simulink model "fuz_model"  (R2018a)
settings: Solver=VariableStepAuto  StartTime=0.0  StopTime=inf  RelTol=1e-3
undefined symbols (not defined in the file): DeltaDVal, DeltaIVal, DeltaPVal
libraries: robotlib x5, fuzblock x1
settings Model: Creator=piradata  LastModifiedBy=piradata
settings DataIOCC: SaveOutput=off  SignalLogging=off  DSMLogging=off  SaveTime=off

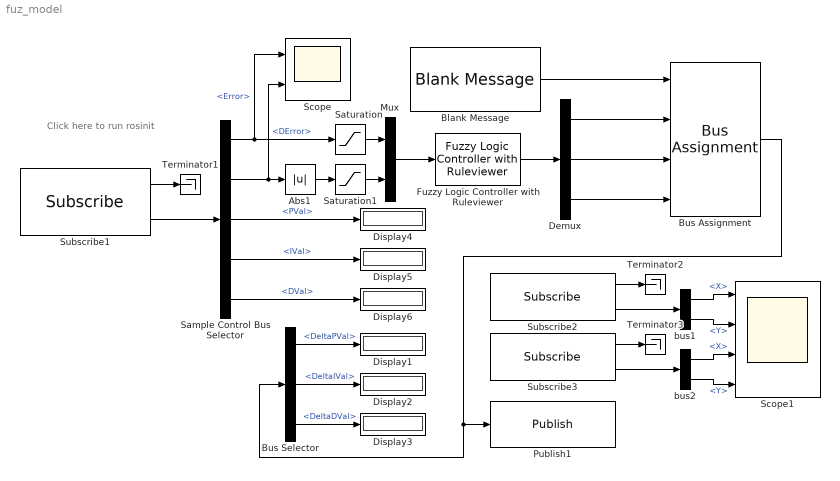
== system fuz_model ==
  note: Click here to run
      | rosinit
  Abs1 : Abs
  Blank Message : robotlib/Blank Message  SourceLibraryInfo=This block requires Robotics System Toolbox  messageType=wpg/defuzzyfied  SampleTime=inf
      settings: SourceProductBaseCode=RO
  Bus Assignment : BusAssignment  AssignedSignals=DeltaPVal,DeltaIVal,DeltaDVal
  Bus Selector : BusSelector  OutputSignals=DeltaPVal,DeltaIVal,DeltaDVal
  Demux : Demux  Outputs=3
  Display{1..6} (6 alike) : Display
  Fuzzy Logic Controller with Ruleviewer : fuzblock/Fuzzy Logic  Controller  with Ruleviewer  fismatrix=Drone2  Ts=2
  Mux : Mux  Inputs=2
  Publish1 : robotlib/Publish  SourceLibraryInfo=This block requires Robotics System Toolbox  topicSource=Specify your own  topic=/defuzzy_values  messageType=wpg/defuzzyfied  messageQueueLength=1
      settings: SourceProductBaseCode=RO
  Sample Control Bus Selector : BusSelector  OutputSignals=Error,DError,PVal,IVal,DVal
  Saturation : Saturate
  Saturation1 : Saturate  UpperLimit=1  LowerLimit=-1
  Scope : Scope  NumInputPorts=2
  Scope1 : Scope  NumInputPorts=4
  Subscribe1 : robotlib/Subscribe  SourceLibraryInfo=This block requires Robotics System Toolbox  topicSource=Specify your own  topic=/fuzzy_values  messageType=wpg/fuzzy  sampleTime=-1  messageQueueLength=1
      settings: SourceProductBaseCode=RO
  Subscribe2 : robotlib/Subscribe  SourceLibraryInfo=This block requires Robotics System Toolbox  topicSource=Select from ROS network  topic=/reference_pos  messageType=geometry_msgs/PoseStamped  sampleTime=-1  messageQueueLength=1
      settings: SourceProductBaseCode=RO
  Subscribe3 : robotlib/Subscribe  SourceLibraryInfo=This block requires Robotics System Toolbox  topicSource=Select from ROS network  topic=/mavros/local_position/pose  messageType=geometry_msgs/PoseStamped  sampleTime=-1  messageQueueLength=1
      settings: SourceProductBaseCode=RO
  Terminator1 : Terminator
  Terminator2 : Terminator
  Terminator3 : Terminator
  bus1 : BusSelector  OutputSignals=Pose.Position.X,Pose.Position.Y
  bus2 : BusSelector  OutputSignals=Pose.Position.X,Pose.Position.Y
  wires:
  Bus Selector/3 -> Display3/1  "<DeltaDVal>"
  Bus Selector/2 -> Display2/1  "<DeltaIVal>"
  Bus Assignment/1 -> Bus Selector/1, Publish1/1
  Bus Selector/1 -> Display1/1  "<DeltaPVal>"
  Blank Message/1 -> Bus Assignment/1
  Subscribe1/1 -> Terminator1/1
  Fuzzy Logic Controller with Ruleviewer/1 -> Demux/1
  Demux/1 -> Bus Assignment/2
  Subscribe1/2 -> Sample Control Bus Selector/1
  Sample Control Bus Selector/1 -> Saturation/1, Scope/1  "<Error>"
  Mux/1 -> Fuzzy Logic Controller with Ruleviewer/1
  Sample Control Bus Selector/3 -> Display4/1  "<PVal>"
  Sample Control Bus Selector/4 -> Display5/1  "<IVal>"
  Sample Control Bus Selector/5 -> Display6/1  "<DVal>"
  Saturation/1 -> Mux/1
  Abs1/1 -> Saturation1/1
  Sample Control Bus Selector/2 -> Scope/2, Abs1/1  "<DError>"
  Saturation1/1 -> Mux/2
  Demux/2 -> Bus Assignment/3
  Demux/3 -> Bus Assignment/4
  Subscribe2/1 -> Terminator2/1
  Subscribe2/2 -> bus1/1
  bus1/2 -> Scope1/2  "<Y>"
  bus1/1 -> Scope1/1  "<X>"
  Subscribe3/1 -> Terminator3/1
  Subscribe3/2 -> bus2/1
  bus2/1 -> Scope1/3  "<X>"
  bus2/2 -> Scope1/4  "<Y>"
